simulink library "csc_mnc_measurement_noise_covariance_lib"  (R2015b)
settings: Solver=VariableStepAuto  StartTime=0.0  StopTime=10.0  RelTol=1e-3
values from neighbouring files (symbols this model uses):
  mnc_meas_noise_indep = [ 9e-4 9e-4 9e-4]    [csc_mnc_measurement_noise_covariance_init.m]
libraries: csc_src_slant_range_covariance_lib x4, util_info_lib x2, csc_hvc_homography_velocity_covariance_lib x2
settings Model: Creator=Mark Agbayani  LastModifiedBy=Mark Agbayani

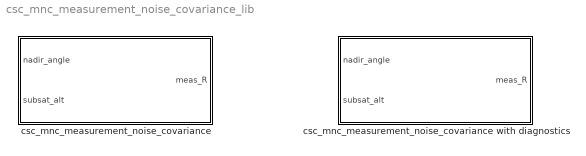
== system csc_mnc_measurement_noise_covariance_lib ==
  csc_mnc_measurement_noise_covariance : Subsystem
  csc_mnc_measurement_noise_covariance with diagnostics : Subsystem

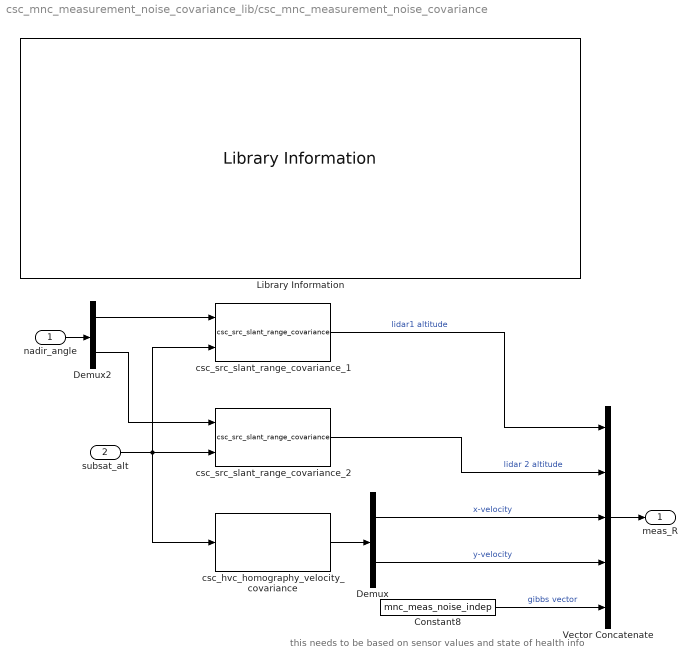
== system csc_mnc_measurement_noise_covariance_lib/csc_mnc_measurement_noise_covariance ==
  note: this needs to be based on sensor values and state of health info
  nadir_angle : Inport
  subsat_alt : Inport  Port=2
  Constant8 : Constant  Value=mnc_meas_noise_indep
  Demux : Demux  Outputs=2
  Demux2 : Demux  Outputs=2
  Library Information : util_info_lib/Library Information  owner='NONE'
  Vector Concatenate : Concatenate  NumInputs=5
  csc_hvc_homography_velocity_covariance : csc_hvc_homography_velocity_covariance_lib/csc_hvc_homography_velocity_covariance
  csc_src_slant_range_covariance_1 : csc_src_slant_range_covariance_lib/csc_src_slant_range_covariance  i=1
  csc_src_slant_range_covariance_2 : csc_src_slant_range_covariance_lib/csc_src_slant_range_covariance  i=2
  meas_R : Outport
  wires:
  subsat_alt/1 -> csc_src_slant_range_covariance_1/2, csc_src_slant_range_covariance_2/2, csc_hvc_homography_velocity_covariance/1
  Demux2/2 -> csc_src_slant_range_covariance_2/1
  Demux2/1 -> csc_src_slant_range_covariance_1/1
  nadir_angle/1 -> Demux2/1
  csc_src_slant_range_covariance_2/1 -> Vector Concatenate/2  "lidar 2 altitude"
  csc_src_slant_range_covariance_1/1 -> Vector Concatenate/1  "lidar1 altitude"
  Vector Concatenate/1 -> meas_R/1
  Constant8/1 -> Vector Concatenate/5  "gibbs vector"
  csc_hvc_homography_velocity_covariance/1 -> Demux/1
  Demux/2 -> Vector Concatenate/4  "y-velocity"
  Demux/1 -> Vector Concatenate/3  "x-velocity"

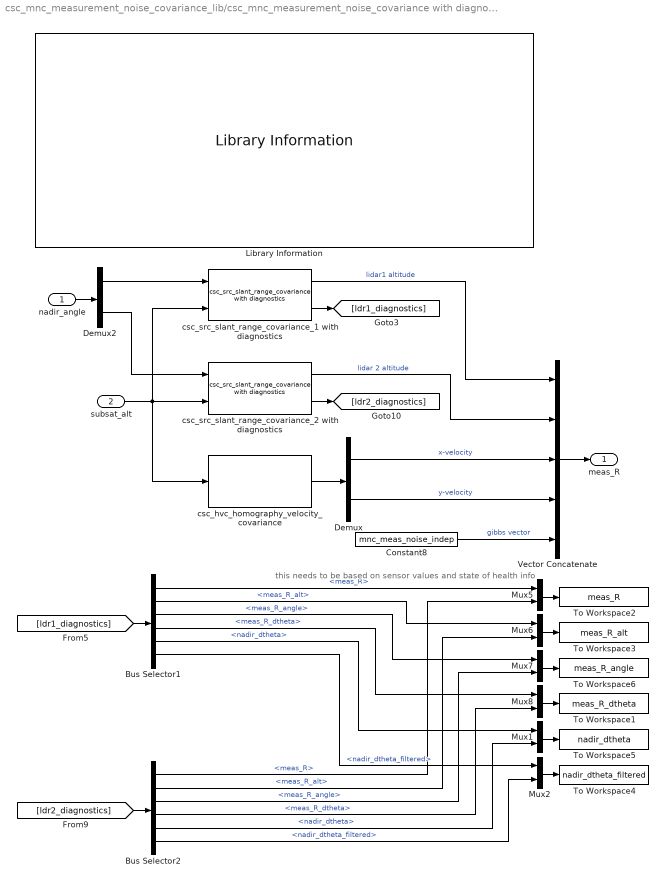
== system csc_mnc_measurement_noise_covariance_lib/csc_mnc_measurement_noise_covariance with diagnostics ==
  note: this needs to be based on sensor values and state of health info
  nadir_angle : Inport
  subsat_alt : Inport  Port=2
  Bus Selector1 : BusSelector  OutputSignals=meas_R,meas_R_alt,meas_R_angle,meas_R_dtheta,nadir_dtheta,nadir_dtheta_filtered
  Bus Selector2 : BusSelector  OutputSignals=meas_R,meas_R_alt,meas_R_angle,meas_R_dtheta,nadir_dtheta,nadir_dtheta_filtered
  Constant8 : Constant  Value=mnc_meas_noise_indep
  Demux : Demux  Outputs=2
  Demux2 : Demux  Outputs=2
  Library Information : util_info_lib/Library Information  owner='NONE'
  Mux{1..2,5..8} (6 alike) : Mux  Inputs=2
  To Workspace1 : ToWorkspace  VariableName=meas_R_dtheta  SaveFormat=Structure With Time  SampleTime=-1
  To Workspace2 : ToWorkspace  VariableName=meas_R  SaveFormat=Structure With Time  SampleTime=-1
  To Workspace3 : ToWorkspace  VariableName=meas_R_alt  SaveFormat=Structure With Time  SampleTime=-1
  To Workspace4 : ToWorkspace  VariableName=nadir_dtheta_filtered  SaveFormat=Structure With Time  SampleTime=-1
  To Workspace5 : ToWorkspace  VariableName=nadir_dtheta  SaveFormat=Structure With Time  SampleTime=-1
  To Workspace6 : ToWorkspace  VariableName=meas_R_angle  SaveFormat=Structure With Time  SampleTime=-1
  Vector Concatenate : Concatenate  NumInputs=5
  csc_hvc_homography_velocity_covariance : csc_hvc_homography_velocity_covariance_lib/csc_hvc_homography_velocity_covariance
  csc_src_slant_range_covariance_1 with diagnostics : csc_src_slant_range_covariance_lib/csc_src_slant_range_covariance with diagnostics  i=1
  csc_src_slant_range_covariance_2 with diagnostics : csc_src_slant_range_covariance_lib/csc_src_slant_range_covariance with diagnostics  i=2
  meas_R : Outport
  wires:
  Mux2/1 -> To Workspace4/1
  Bus Selector2/6 -> Mux2/2  "<nadir_dtheta_filtered>"
  Bus Selector2/5 -> Mux1/2  "<nadir_dtheta>"
  Mux1/1 -> To Workspace5/1
  subsat_alt/1 -> csc_src_slant_range_covariance_2 with diagnostics/2, csc_hvc_homography_velocity_covariance/1, csc_src_slant_range_covariance_1 with diagnostics/2
  csc_src_slant_range_covariance_1 with diagnostics/2 -> [ldr1_diagnostics]
  Bus Selector1/6 -> Mux2/1  "<nadir_dtheta_filtered>"
  csc_src_slant_range_covariance_2 with diagnostics/2 -> [ldr2_diagnostics]
  Bus Selector2/4 -> Mux8/2  "<meas_R_dtheta>"
  Bus Selector1/4 -> Mux8/1  "<meas_R_dtheta>"
  Bus Selector2/3 -> Mux7/2  "<meas_R_angle>"
  Bus Selector1/3 -> Mux7/1  "<meas_R_angle>"
  Bus Selector2/2 -> Mux6/2  "<meas_R_alt>"
  Bus Selector1/2 -> Mux6/1  "<meas_R_alt>"
  Bus Selector2/1 -> Mux5/2  "<meas_R>"
  Bus Selector1/1 -> Mux5/1  "<meas_R>"
  [ldr1_diagnostics] -> Bus Selector1/1
  [ldr2_diagnostics] -> Bus Selector2/1
  Bus Selector1/5 -> Mux1/1  "<nadir_dtheta>"
  Mux8/1 -> To Workspace1/1
  Mux7/1 -> To Workspace6/1
  Mux6/1 -> To Workspace3/1
  Mux5/1 -> To Workspace2/1
  Demux2/2 -> csc_src_slant_range_covariance_2 with diagnostics/1
  Demux2/1 -> csc_src_slant_range_covariance_1 with diagnostics/1
  nadir_angle/1 -> Demux2/1
  csc_src_slant_range_covariance_2 with diagnostics/1 -> Vector Concatenate/2  "lidar 2 altitude"
  csc_src_slant_range_covariance_1 with diagnostics/1 -> Vector Concatenate/1  "lidar1 altitude"
  Vector Concatenate/1 -> meas_R/1
  Constant8/1 -> Vector Concatenate/5  "gibbs vector"
  csc_hvc_homography_velocity_covariance/1 -> Demux/1
  Demux/2 -> Vector Concatenate/4  "y-velocity"
  Demux/1 -> Vector Concatenate/3  "x-velocity"
